simulink model "model_neliniar_reactoare"  (R2023b)
settings: Solver=VariableStepAuto  StartTime=0.0  StopTime=10  RelTol=1e-3
undefined symbols (not defined in the file or in its folder): c0, ci, EdR, hA, k0, mdH, q, rcp, T0, Ti, Tr, V
settings Model: Creator=domid  LastModifiedBy=domid

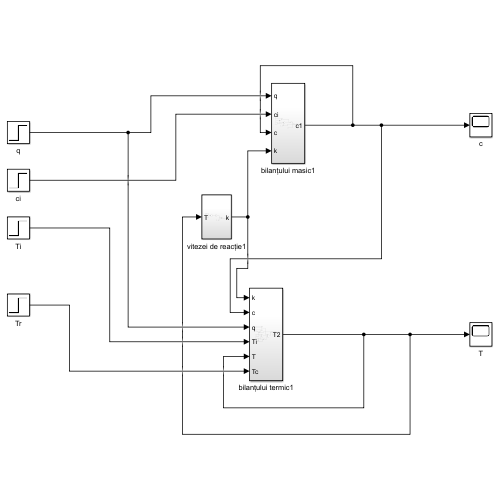
[thumbnail: Simulink's stored preview of the top-level diagram]
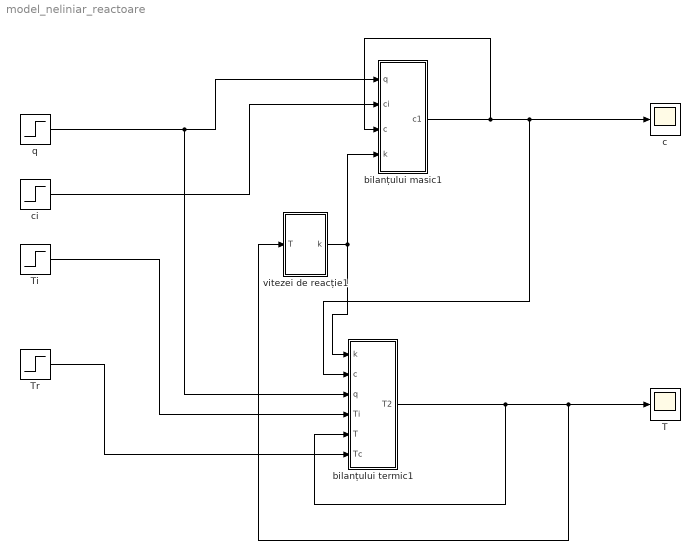
== system model_neliniar_reactoare ==
  T : Scope
  Ti : Step  Time=0  Before=Ti  After=Ti  SampleTime=0
  Tr : Step  Time=0  Before=Tr  After=Tr  SampleTime=0
  bilanțului masic1 : Subsystem
  bilanțului termic1 : Subsystem
  c : Scope
  ci : Step  Time=0  Before=ci  After=ci  SampleTime=0
  q : Step  Time=0  Before=q  After=q  SampleTime=0
  vitezei de reacție1 : Subsystem
  wires:
  q/1 -> bilanțului masic1/1(q), bilanțului termic1/3(q)
  ci/1 -> bilanțului masic1/2(ci)
  Ti/1 -> bilanțului termic1/4(Ti)
  Tr/1 -> bilanțului termic1/6(Tc)
  bilanțului termic1/1(T2) -> bilanțului termic1/5(T), vitezei de reacție1/1(T), T/1
  bilanțului masic1/1(c1) -> bilanțului masic1/3(c), bilanțului termic1/2(c), c/1
  vitezei de reacție1/1(k) -> bilanțului termic1/1(k), bilanțului masic1/4(k)

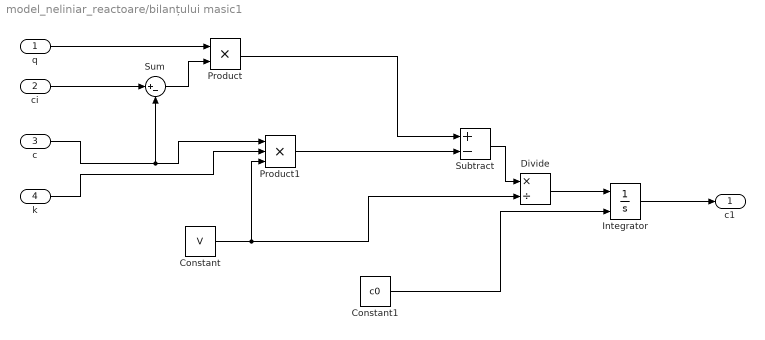
== system model_neliniar_reactoare/bilanțului masic1 ==
  q : Inport
  ci : Inport  Port=2
  c : Inport  Port=3
  k : Inport  Port=4
  Constant : Constant  Value=V
  Constant1 : Constant  Value=c0
  Divide : Product  Inputs=*/
  Integrator : Integrator  InitialConditionSource=external
  Product : Product
  Product1 : Product  Inputs=3
  Subtract : Sum  Inputs=+-
  Sum : Sum  Inputs=|+-
  c1 : Outport
  wires:
  Subtract/1 -> Divide/1
  q/1 -> Product/1
  Product/1 -> Subtract/1
  Constant/1 -> Product1/3, Divide/2
  Product1/1 -> Subtract/2
  k/1 -> Product1/2
  Divide/1 -> Integrator/1
  ci/1 -> Sum/1
  Sum/1 -> Product/2
  c/1 -> Sum/2, Product1/1
  Integrator/1 -> c1/1
  Constant1/1 -> Integrator/2

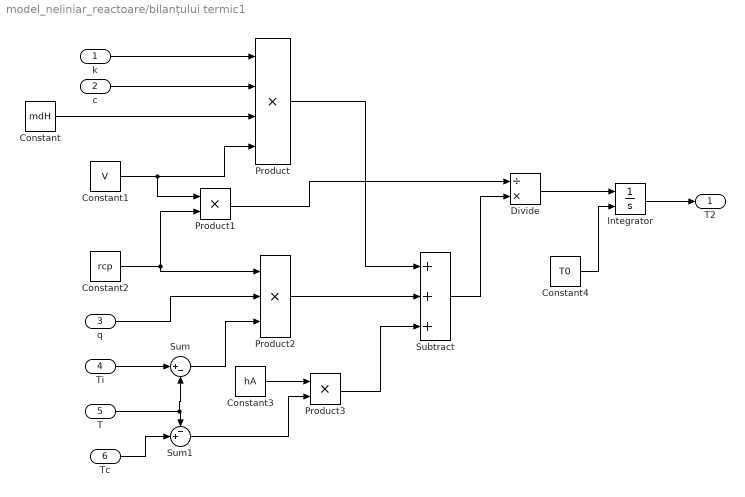
== system model_neliniar_reactoare/bilanțului termic1 ==
  k : Inport
  c : Inport  Port=2
  q : Inport  Port=3
  Ti : Inport  Port=4
  T : Inport  Port=5
  Tc : Inport  Port=6
  Constant : Constant  Value=mdH
  Constant1 : Constant  Value=V
  Constant2 : Constant  Value=rcp
  Constant3 : Constant  Value=hA
  Constant4 : Constant  Value=T0
  Divide : Product  Inputs=/*
  Integrator : Integrator  InitialConditionSource=external
  Product : Product  Inputs=4
  Product1 : Product
  Product2 : Product  Inputs=3
  Product3 : Product
  Subtract : Sum  Inputs=+++
  Sum : Sum  Inputs=|+-
  Sum1 : Sum  Inputs=-+|
  T2 : Outport
  wires:
  Sum1/1 -> Product3/2
  q/1 -> Product2/2
  T/1 -> Sum/2, Sum1/1
  Product/1 -> Subtract/1
  Constant1/1 -> Product1/1, Product/4
  c/1 -> Product/2
  Constant4/1 -> Integrator/2
  Constant2/1 -> Product2/1, Product1/2
  k/1 -> Product/1
  Tc/1 -> Sum1/2
  Ti/1 -> Sum/1
  Constant/1 -> Product/3
  Sum/1 -> Product2/3
  Constant3/1 -> Product3/1
  Divide/1 -> Integrator/1
  Subtract/1 -> Divide/2
  Product1/1 -> Divide/1
  Product3/1 -> Subtract/3
  Integrator/1 -> T2/1
  Product2/1 -> Subtract/2

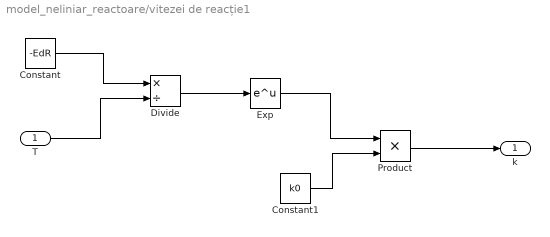
== system model_neliniar_reactoare/vitezei de reacție1 ==
  T : Inport
  Constant : Constant  Value=-EdR
  Constant1 : Constant  Value=k0
  Divide : Product  Inputs=*/
  Exp : Math
  Product : Product
  k : Outport
  wires:
  Constant1/1 -> Product/2
  Constant/1 -> Divide/1
  Product/1 -> k/1
  T/1 -> Divide/2
  Exp/1 -> Product/1
  Divide/1 -> Exp/1
